simulink model "peacockElettricaSimulink2025b"  (R2025b)
settings: Solver=FixedStepAuto  StopTime=30  FixedStep=0.001  MaxStep=0.001
InitFcn:
  | run('setupParams.m');
StopFcn:
  | plot(out.X, out.Y); axis equal; grid on;
model workspace: external: MATLAB File (data not in the file)
values from neighbouring files (symbols this model uses):
  air_temp = 300    [setupParams.m]    (also in setupParamsSingle.m)
  brake_bias_f = 0.60    (= 0.6)    [setupParams.m]    (also in setupParamsSingle.m)
  brake_bias_r = 1 - brake_bias_f    (= 0.4)    [setupParams.m]    (also in setupParamsSingle.m)
  camber_front = -1.5    [setupParams.m]    (also in setupParamsSingle.m)
  camber_rear = -1    [setupParams.m]    (also in setupParamsSingle.m)
  g = 9.81    [setupParams.m]    (also in setupParamsSingle.m)
  gnd_displ = 0.0    (= 0)    [setupParams.m]    (also in setupParamsSingle.m)
  Kus = 0.00    (= 0)    [setupParams.m]    (also in setupParamsSingle.m)
  l_f = 0.775    [setupParams.m]    (also in setupParamsSingle.m)
  l_r = 0.775    [setupParams.m]    (also in setupParamsSingle.m)
  launch_ramp_rate = 1000.0    (= 1000)    [setupParams.m]    (also in setupParamsSingle.m)
  launch_V_thresh = 5.0    (= 5)    [setupParams.m]    (also in setupParamsSingle.m)
  mass = 300    [setupParams.m]    (also in setupParamsSingle.m)
  mu = 1.5    [setupParams.m]    (also in setupParamsSingle.m)
  nominal_ramp_rate = 1000.0    (= 1000)    [setupParams.m]    (also in setupParamsSingle.m)
  pa_front_wheel = 82700    [setupParams.m]    (also in setupParamsSingle.m)
  pa_rear_wheel = 82700    [setupParams.m]    (also in setupParamsSingle.m)
  pedal_bp = (0:10:100)'    [setupParams.m]    (also in setupParamsSingle.m)
  pedal_map = (pedal_bp / 100) .^ pedal_alpha    [setupParams.m]    (also in setupParamsSingle.m = (pedal_bp / 100) .^ pedal_alpha.Value)
  R_wheel = 0.2032    [setupParams.m]    (also in setupParamsSingle.m)
  regen_I_cont_A = 14.0    (= 14)    [setupParams.m]    (also in setupParamsSingle.m)
  regen_I_peak_A = 21.0    (= 21)    [setupParams.m]    (also in setupParamsSingle.m)
  regen_I_peak_dur_s = 4.0    (= 4)    [setupParams.m]    (also in setupParamsSingle.m)
  regen_P_batt_max_W = 35000    [setupParams.m]    (also in setupParamsSingle.m)
  regen_pedal_thr = 10.0    (= 10)    [setupParams.m]    (also in setupParamsSingle.m)
  regen_speed_crit_rpm = 2000    [setupParams.m]    (also in setupParamsSingle.m = 500)
  regen_speed_min_rpm = 4000    [setupParams.m]    (also in setupParamsSingle.m = 3000)
  regen_T_max = 5    [setupParams.m]    (also in setupParamsSingle.m = Simulink.Parameter(T_rated.Value/2))
  rid_eff = 0.80    (= 0.8)    [setupParams.m]    (also in setupParamsSingle.m)
  rid_ratio = 15    [setupParams.m]    (also in setupParamsSingle.m)
  scale_factor_front = ones(27, 1)    [setupParams.m]    (also in setupParamsSingle.m)
  scale_factor_rear = ones(27, 1)    [setupParams.m]    (also in setupParamsSingle.m)
  slc_Ki = 0    [setupParams.m]    (also in setupParamsSingle.m = Simulink.Parameter(0))
  slc_Kp = 0    [setupParams.m]    (also in setupParamsSingle.m = Simulink.Parameter(0))
  slc_low_sat = -T_peak    (= -21)    [setupParams.m]    (also in setupParamsSingle.m)
  slc_up_sat = T_peak    (= 21)    [setupParams.m]    (also in setupParamsSingle.m)
  slip_bc_coeff = 10    [setupParams.m]    (also in setupParamsSingle.m = Simulink.Parameter(1.5))
  slip_filt_N = 80    [setupParams.m]    (also in setupParamsSingle.m = 15)
  slip_Kd = 0.8    [setupParams.m]    (also in setupParamsSingle.m = Simulink.Parameter(5.0))
  slip_Ki = 13.0    (= 13)    [setupParams.m]    (also in setupParamsSingle.m = Simulink.Parameter(110.0))
  slip_Kp = 50.0    (= 50)    [setupParams.m]    (also in setupParamsSingle.m = Simulink.Parameter(180.0))
  slip_low_sat = 0.0    (= 0)    [setupParams.m]    (also in setupParamsSingle.m)
  slip_ref = 0.15    [setupParams.m]    (also in setupParamsSingle.m = Simulink.Parameter(0.15))
  slip_up_sat = 18    [setupParams.m]    (also in setupParamsSingle.m = 21)
  slip_V_min = 3    [setupParams.m]    (also in setupParamsSingle.m = 1)
  steer_ratio = 4.2    [pure_pursuit.m]    (also in setupParams.m; setupParamsSingle.m)
  T_headroom_max = 3.0    (= 3)    [setupParams.m]    (also in setupParamsSingle.m = Simulink.Parameter(5.0))
  T_peak = 21    [setupParams.m]    (also in setupParamsSingle.m)
  T_rated = 9.8    [setupParams.m]    (also in setupParamsSingle.m = Simulink.Parameter(9.8))
  track_width = (track_width_r + track_width_f)/2    (= 1.2)    [setupParams.m]    (also in setupParamsSingle.m = sqrt(track_width_r^2 + track_width_f^2))
  track_width_f = 1.2    [setupParams.m]    (also in setupParamsSingle.m)
  track_width_r = 1.2    [setupParams.m]    (also in setupParamsSingle.m)
  Ts = 0.01    [setupParams.m]    (also in setupParamsSingle.m)
  tvc_D_thresh = 0.060    (= 0.06)    [setupParams.m]    (also in setupParamsSingle.m)
  tvc_D_thresh_off = 0.03    [setupParams.m]    (also in setupParamsSingle.m)
  tvc_Kd = 8    [setupParams.m]    (also in setupParamsSingle.m = Simulink.Parameter(5))
  tvc_Ki = 250    [setupParams.m]    (also in setupParamsSingle.m = Simulink.Parameter(10))
  tvc_Kp = 650    [setupParams.m]    (also in setupParamsSingle.m = Simulink.Parameter(70))
  tvc_low_sat = Simulink.Parameter(0)    [setupParamsSingle.m]
  tvc_throttle_on = 3.0    (= 3)    [setupParams.m]    (also in setupParamsSingle.m = Simulink.Parameter(3.0))
  tvc_up_sat = Simulink.Parameter(T_peak)    [setupParamsSingle.m]
  tvc_V_off = 2.0    (= 2)    [setupParams.m]    (also in setupParamsSingle.m = Simulink.Parameter(2.0))
  tvc_V_on = 4.0    (= 4)    [setupParams.m]    (also in setupParamsSingle.m = Simulink.Parameter(4.0))
  tvc_yaw_thresh = 0.08    [setupParams.m]    (also in setupParamsSingle.m)
  tvc_yaw_thresh_off = 0.04    [setupParams.m]    (also in setupParamsSingle.m)
  v0_speed = 0.00    (= 0)    [setupParams.m]    (also in setupParamsSingle.m)
  V_dc = 540    [setupParams.m]    (also in setupParamsSingle.m)
  w_engine = 0.005    [setupParams.m]    (also in setupParamsSingle.m)
  wheelbase = l_f + l_r    (= 1.55)    [setupParams.m]    (also in setupParamsSingle.m)
libraries: simulink x12, slpidlib x4, vehdynlibtire x4, vehdynlibsteering x1, sim3dlib x1, sim3dautolib x1, autolibshared x1
(part 2 of 3)

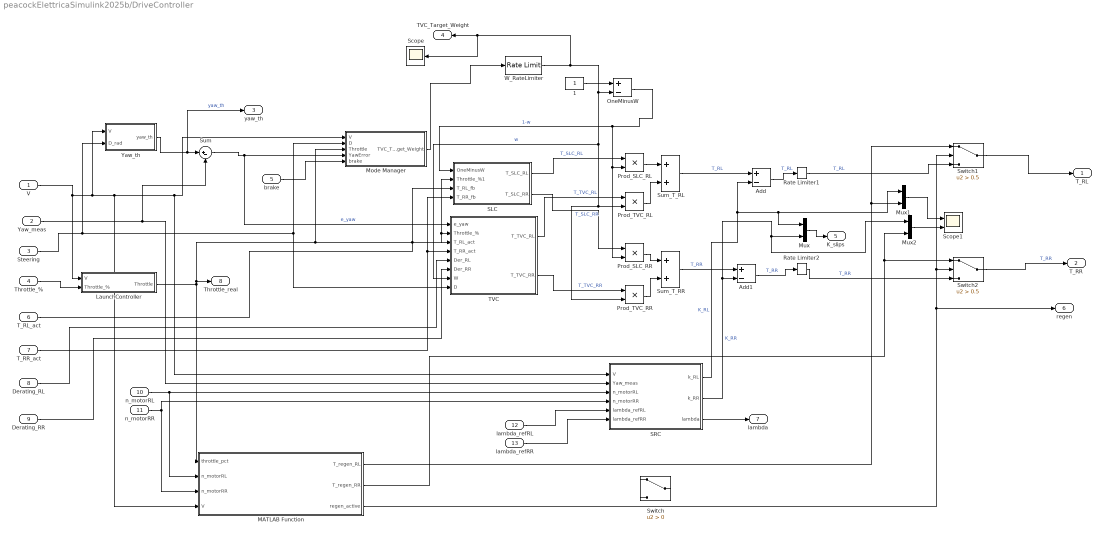
== system peacockElettricaSimulink2025b/DriveController ==
  V : Inport
  Yaw_meas : Inport  Port=2
  Steering : Inport  Port=3
  Throttle_% : Inport  Port=4
  brake : Inport  Port=5
  T_RL_act : Inport  Port=6
  T_RR_act : Inport  Port=7
  Derating_RL : Inport  Port=8
  Derating_RR : Inport  Port=9
  n_motorRL : Inport  Port=10
  n_motorRR : Inport  Port=11
  lambda_refRL : Inport  Port=12
  lambda_refRR : Inport  Port=13
  1 : Constant
  Add : Sum  Inputs=+-
  Add1 : Sum  Inputs=+-
  LaunchController : Subsystem
  MATLAB Function : MATLAB Function  TreatAsAtomicUnit=on
  Mode Manager : Stateflow chart  TreatAsAtomicUnit=on
  Mux : Mux  Inputs=2
  Mux1 : Mux  Inputs=2
  Mux2 : Mux  Inputs=2
  OneMinusW : Sum  Inputs=+-
  Prod_SLC_RL : Product  Inputs=**
  Prod_SLC_RR : Product  Inputs=**
  Prod_TVC_RL : Product  Inputs=**
  Prod_TVC_RR : Product  Inputs=**
  Rate Limiter1 : RateLimiter  RisingSlewLimit=18  FallingSlewLimit=-21  SampleTimeMode=inherited
  Rate Limiter2 : RateLimiter  RisingSlewLimit=18  FallingSlewLimit=-21  SampleTimeMode=inherited
  SLC : Subsystem  TreatAsAtomicUnit=on
  SRC : Subsystem
  Scope : Scope
      settings: ActiveDisplayYMinimum=0.75000000000000011  ActiveDisplayYMaximum=3.25  DataLoggingVariableName=ScopeData5
  Scope1 : Scope  NumInputPorts=2
      settings: ActiveDisplayYMinimum=-0.12499999999999997  ActiveDisplayYMaximum=1.125  DataLoggingVariableName=ScopeData7
  Sum : Sum  Inputs=|+-
  Sum_T_RL : Sum
  Sum_T_RR : Sum
  Switch : Switch  Criteria=u2 > Threshold  SaturateOnIntegerOverflow=off  InputSameDT=off
  Switch1 : Switch  Criteria=u2 > Threshold  Threshold=0.5  SaturateOnIntegerOverflow=off  InputSameDT=off
  Switch2 : Switch  Criteria=u2 > Threshold  Threshold=0.5  SaturateOnIntegerOverflow=off  InputSameDT=off
  TVC : Subsystem
  W_RateLimiter : RateLimiter  RisingSlewLimit=2  FallingSlewLimit=-2  SampleTimeMode=inherited
  Yaw_th : Subsystem
  T_RL : Outport
  T_RR : Outport  Port=2
  yaw_th : Outport  Port=3
  TVC_Target_Weight : Outport  Port=4
  K_slips : Outport  Port=5
  regen : Outport  Port=6
  lambda : Outport  Port=7
  Throttle_real : Outport  Port=8
  wires:
  Steering/1 -> TVC/8(D), Mode Manager/2(D), Yaw_th/2(D_rad)
  Yaw_th/1(yaw_th) -> yaw_th/1, Sum/1  "yaw_th"
  Derating_RL/1 -> TVC/5(Der_RL)
  Yaw_meas/1 -> SRC/2(Yaw_meas), Sum/2
  Derating_RR/1 -> TVC/6(Der_RR)
  LaunchController/1(Throttle) -> Throttle_real/1, Mode Manager/3(Throttle), SLC/2(Throttle_%1), TVC/2(Throttle_%), MATLAB Function/1(throttle_pct)
  TVC/2(T_TVC_RR) -> Prod_TVC_RR/1  "T_TVC_RR"
  V/1 -> LaunchController/1(V), MATLAB Function/4(V), SRC/1(V), Mode Manager/1(V), Yaw_th/1(V)
  T_RL_act/1 -> SLC/3(T_RL_fb), TVC/3(T_RL_act)
  T_RR_act/1 -> SLC/4(T_RR_fb), TVC/4(T_RR_act)
  TVC/1(T_TVC_RL) -> Prod_TVC_RL/1  "T_TVC_RL"
  SLC/1(T_SLC_RL) -> Prod_SLC_RL/1  "T_SLC_RL"
  SLC/2(T_SLC_RR) -> Prod_SLC_RR/1  "T_SLC_RR"
  brake/1 -> Mode Manager/5(brake)
  Sum/1 -> TVC/1(e_yaw), Mode Manager/4(YawError)  "e_yaw"
  W_RateLimiter/1 -> Scope/1, TVC_Target_Weight/1, Prod_TVC_RR/2, Prod_TVC_RL/2, TVC/7(W), OneMinusW/2  "w"
  1/1 -> OneMinusW/1
  OneMinusW/1 -> Prod_SLC_RL/2, Prod_SLC_RR/2, SLC/1(OneMinusW)  "1-w"
  Prod_SLC_RL/1 -> Sum_T_RL/1
  Prod_TVC_RL/1 -> Sum_T_RL/2
  Prod_SLC_RR/1 -> Sum_T_RR/1
  Prod_TVC_RR/1 -> Sum_T_RR/2
  Mode Manager/1(TVC_Target_Weight) -> W_RateLimiter/1
  Add/1 -> Rate Limiter1/1  "T_RL"
  Sum_T_RR/1 -> Add1/1  "T_RR"
  Rate Limiter1/1 -> Switch1/3  "T_RL"
  Add1/1 -> Rate Limiter2/1  "T_RR"
  n_motorRL/1 -> SRC/3(n_motorRL), MATLAB Function/2(n_motorRL)
  n_motorRR/1 -> SRC/4(n_motorRR), MATLAB Function/3(n_motorRR)
  lambda_refRL/1 -> SRC/5(lambda_refRL)
  lambda_refRR/1 -> SRC/6(lambda_refRR)
  SRC/1(k_RL) -> Add/2, Mux/1, Mux1/1  "K_RL"
  SRC/2(k_RR) -> Add1/2, Mux2/1, Mux/2  "K_RR"
  Switch2/1 -> T_RR/1  "T_RR"
  Sum_T_RL/1 -> Add/1  "T_RL"
  Mux/1 -> K_slips/1
  MATLAB Function/2(T_regen_RR) -> Mux2/2, Switch2/1
  MATLAB Function/1(T_regen_RL) -> Switch1/1, Mux1/2
  Mux1/1 -> Scope1/1
  Mux2/1 -> Scope1/2
  MATLAB Function/3(regen_active) -> regen/1, Switch1/2, Switch2/2
  Switch1/1 -> T_RL/1
  Rate Limiter2/1 -> Switch2/3  "T_RR"
  Throttle_%/1 -> LaunchController/2(Throttle_%)
  SRC/3(lambda) -> lambda/1

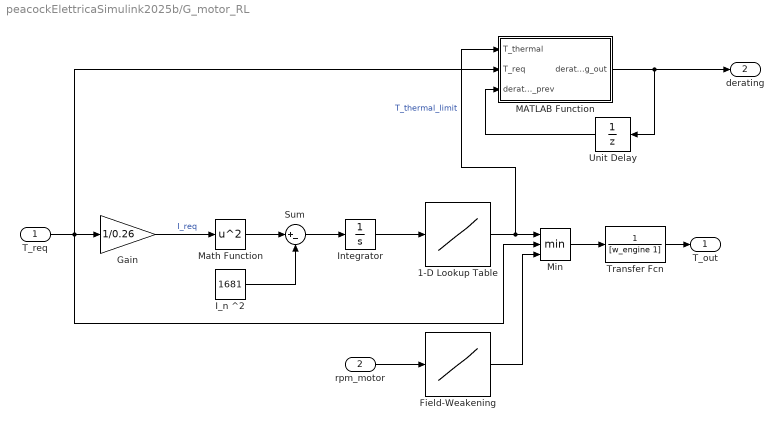
== system peacockElettricaSimulink2025b/G_motor_RL ==
  T_req : Inport
  rpm_motor : Inport  Port=2
  1-D Lookup Table : Lookup_n-D  NumberOfTableDimensions=1  BreakpointsForDimension1=[0, 9268, 11586.6]  Table=[21, 21, 9.8]  InternalRulePriority=Speed  RndMeth=Simplest
  Field-Weakening : Lookup_n-D  NumberOfTableDimensions=1  BreakpointsForDimension1=[0, 12000, 14000, 16000, 18000, 20000]  Table=[21, 21, 20, 16, 9, 0]  InternalRulePriority=Speed  RndMeth=Simplest
  Gain : Gain  Gain=1/0.26
  I_n ^2 : Constant  Value=1681
  Integrator : Integrator  LimitOutput=on  UpperSaturationLimit=11586.6  LowerSaturationLimit=0
  MATLAB Function : MATLAB Function  TreatAsAtomicUnit=on
  Math Function : Math  Operator=square
  Min : MinMax  Inputs=3
  Sum : Sum  Inputs=|+-
  Transfer Fcn : TransferFcn  Denominator=[w_engine 1]
  Unit Delay : UnitDelay  SampleTime=-1
  T_out : Outport
  derating : Outport  Port=2
  wires:
  Sum/1 -> Integrator/1
  I_n ^2/1 -> Sum/2
  Gain/1 -> Math Function/1  "I_req"
  Math Function/1 -> Sum/1
  Integrator/1 -> 1-D Lookup Table/1
  Min/1 -> Transfer Fcn/1
  Transfer Fcn/1 -> T_out/1
  1-D Lookup Table/1 -> MATLAB Function/1(T_thermal), Min/1  "T_thermal_limit"
  T_req/1 -> MATLAB Function/2(T_req), Min/2, Gain/1
  MATLAB Function/1(derating_out) -> Unit Delay/1, derating/1
  Unit Delay/1 -> MATLAB Function/3(derating_prev)
  rpm_motor/1 -> Field-Weakening/1
  Field-Weakening/1 -> Min/3

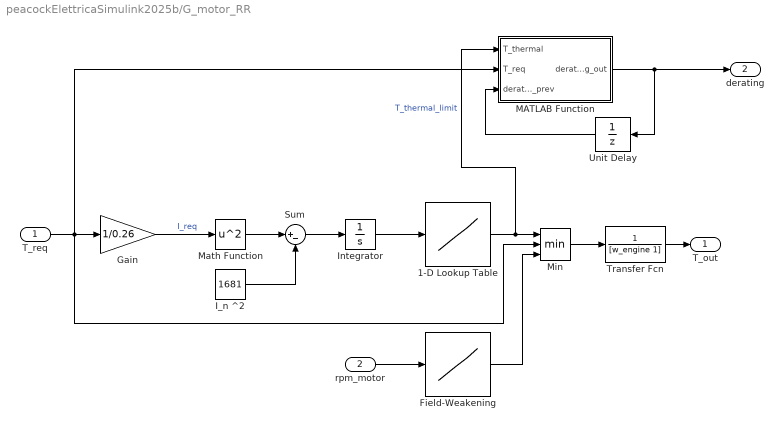
== system peacockElettricaSimulink2025b/G_motor_RR ==
  T_req : Inport
  rpm_motor : Inport  Port=2
  1-D Lookup Table : Lookup_n-D  NumberOfTableDimensions=1  BreakpointsForDimension1=[0, 9268, 11586.6]  Table=[21, 21, 9.8]  InternalRulePriority=Speed  RndMeth=Simplest
  Field-Weakening : Lookup_n-D  NumberOfTableDimensions=1  BreakpointsForDimension1=[0, 12000, 14000, 16000, 18000, 20000]  Table=[21, 21, 20, 16, 9, 0]  InternalRulePriority=Speed  RndMeth=Simplest
  Gain : Gain  Gain=1/0.26
  I_n ^2 : Constant  Value=1681
  Integrator : Integrator  LimitOutput=on  UpperSaturationLimit=11586.6  LowerSaturationLimit=0
  MATLAB Function : MATLAB Function  TreatAsAtomicUnit=on
  Math Function : Math  Operator=square
  Min : MinMax  Inputs=3
  Sum : Sum  Inputs=|+-
  Transfer Fcn : TransferFcn  Denominator=[w_engine 1]
  Unit Delay : UnitDelay  SampleTime=-1
  T_out : Outport
  derating : Outport  Port=2
  wires:
  Sum/1 -> Integrator/1
  I_n ^2/1 -> Sum/2
  Gain/1 -> Math Function/1  "I_req"
  Math Function/1 -> Sum/1
  Integrator/1 -> 1-D Lookup Table/1
  Min/1 -> Transfer Fcn/1
  Transfer Fcn/1 -> T_out/1
  1-D Lookup Table/1 -> MATLAB Function/1(T_thermal), Min/1  "T_thermal_limit"
  T_req/1 -> MATLAB Function/2(T_req), Min/2, Gain/1
  MATLAB Function/1(derating_out) -> Unit Delay/1, derating/1
  Unit Delay/1 -> MATLAB Function/3(derating_prev)
  rpm_motor/1 -> Field-Weakening/1
  Field-Weakening/1 -> Min/3

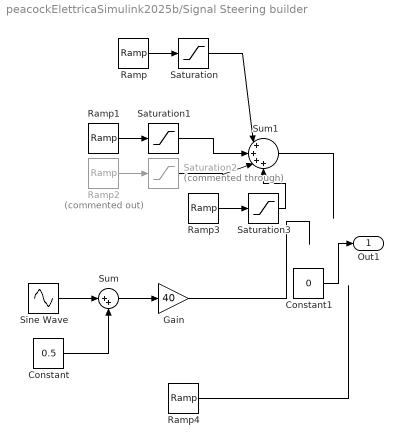
== system peacockElettricaSimulink2025b/Signal Steering builder ==
  Constant : Constant  Value=0.5
  Constant1 : Constant  Value=0
  Gain : Gain  Gain=40
  Ramp : simulink/Sources/Ramp  slope=20  start=0  InitialOutput=0
  Ramp1 : simulink/Sources/Ramp  slope=-20  start=30  InitialOutput=0
  Ramp2 : simulink/Sources/Ramp  Commented=on  slope=-20  start=14  InitialOutput=0
  Ramp3 : simulink/Sources/Ramp  slope=20  start=22  InitialOutput=0
  Ramp4 : simulink/Sources/Ramp  slope=30  start=4  InitialOutput=0
  Saturation : Saturate  UpperLimit=40  LowerLimit=-40
  Saturation1 : Saturate  UpperLimit=40  LowerLimit=-40
  Saturation2 : Saturate  Commented=through  UpperLimit=40  LowerLimit=-40
  Saturation3 : Saturate  UpperLimit=40  LowerLimit=-40
  Sine Wave : Sin  Amplitude=0.5  Frequency=0.3  SampleTime=0.2
  Sum : Sum  Inputs=|++
  Sum1 : Sum  Inputs=|++++
  Out1 : Outport
  wires:
  Ramp/1 -> Saturation/1
  Ramp1/1 -> Saturation1/1
  Ramp2/1 -> Saturation2/1
  Ramp3/1 -> Saturation3/1
  Saturation3/1 -> Sum1/4
  Saturation/1 -> Sum1/1
  Saturation1/1 -> Sum1/2
  Saturation2/1 -> Sum1/3
  Sum1/1 -> ?
  Constant/1 -> Sum/2
  Sine Wave/1 -> Sum/1
  Sum/1 -> Gain/1
  Gain/1 -> ?
  Ramp4/1 -> ?
  Constant1/1 -> Out1/1

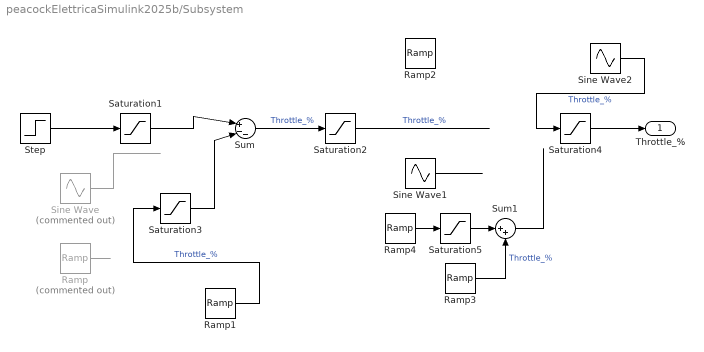
== system peacockElettricaSimulink2025b/Subsystem ==
  Ramp : simulink/Sources/Ramp  Commented=on  slope=1  start=0  InitialOutput=0
  Ramp1 : simulink/Sources/Ramp  slope=40  start=10  InitialOutput=0
  Ramp2 : simulink/Sources/Ramp  slope=100  start=2  InitialOutput=0
  Ramp3 : simulink/Sources/Ramp  slope=50  start=2  InitialOutput=0
  Ramp4 : simulink/Sources/Ramp  slope=50  start=0  InitialOutput=0
  Saturation1 : Saturate  UpperLimit=100  LowerLimit=0
  Saturation2 : Saturate  UpperLimit=100  LowerLimit=0
  Saturation3 : Saturate  UpperLimit=40  LowerLimit=0
  Saturation4 : Saturate  UpperLimit=100  LowerLimit=0
  Saturation5 : Saturate  UpperLimit=60  LowerLimit=0
  Sine Wave : Sin  Commented=on  Amplitude=150  Frequency=0.5  SampleTime=0.2
  Sine Wave1 : Sin  Amplitude=30  Frequency=4  SampleTime=0.01
  Sine Wave2 : Sin  Amplitude=800  Frequency=0.3  SampleTime=Ts
  Step : Step  After=100  SampleTime=0
  Sum : Sum  Inputs=|+--
  Sum1 : Sum  Inputs=|++
  Throttle_% : Outport
  wires:
  Step/1 -> Saturation1/1
  Sine Wave/1 -> ?
  Ramp1/1 -> Saturation3/1  "Throttle_%"
  Ramp/1 -> ?
  Saturation1/1 -> Sum/1
  Saturation3/1 -> Sum/2
  Sum/1 -> Saturation2/1  "Throttle_%"
  Sine Wave2/1 -> Saturation4/1  "Throttle_%"
  Saturation2/1 -> ?  "Throttle_%"
  Ramp3/1 -> Sum1/2  "Throttle_%"
  Sine Wave1/1 -> ?
  Sum1/1 -> ?
  Ramp4/1 -> Saturation5/1
  Saturation4/1 -> Throttle_%/1
  Saturation5/1 -> Sum1/1

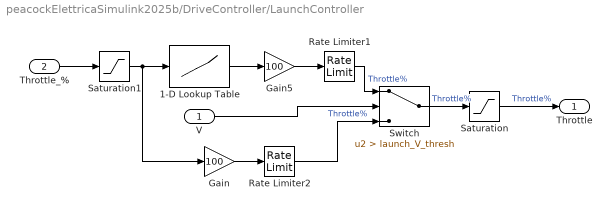
== system peacockElettricaSimulink2025b/DriveController/LaunchController ==
  V : Inport
  Throttle_% : Inport  Port=2
  1-D Lookup Table : Lookup_n-D  NumberOfTableDimensions=1  BreakpointsForDimension1=pedal_bp  Table=pedal_map  ExtrapMethod=Clip  UseLastTableValue=on  InternalRulePriority=Speed  RndMeth=Simplest
  Gain : Gain  Gain=100
  Gain5 : Gain  Gain=100
  Rate Limiter1 : RateLimiter  RisingSlewLimit=launch_ramp_rate  FallingSlewLimit=-100  SampleTimeMode=inherited
  Rate Limiter2 : RateLimiter  RisingSlewLimit=nominal_ramp_rate  FallingSlewLimit=-100  SampleTimeMode=inherited
  Saturation : Saturate  UpperLimit=100  LowerLimit=0
  Saturation1 : Saturate  UpperLimit=100  LowerLimit=0
  Switch : Switch  Criteria=u2 > Threshold  Threshold=launch_V_thresh  SaturateOnIntegerOverflow=off  InputSameDT=off
  Throttle : Outport
  wires:
  Throttle_%/1 -> Saturation1/1
  Saturation1/1 -> Gain/1, 1-D Lookup Table/1
  1-D Lookup Table/1 -> Gain5/1
  Gain5/1 -> Rate Limiter1/1
  Saturation/1 -> Throttle/1  "Throttle%"
  Gain/1 -> Rate Limiter2/1
  Rate Limiter2/1 -> Switch/3  "Throttle%"
  Rate Limiter1/1 -> Switch/1  "Throttle%"
  V/1 -> Switch/2
  Switch/1 -> Saturation/1  "Throttle%"

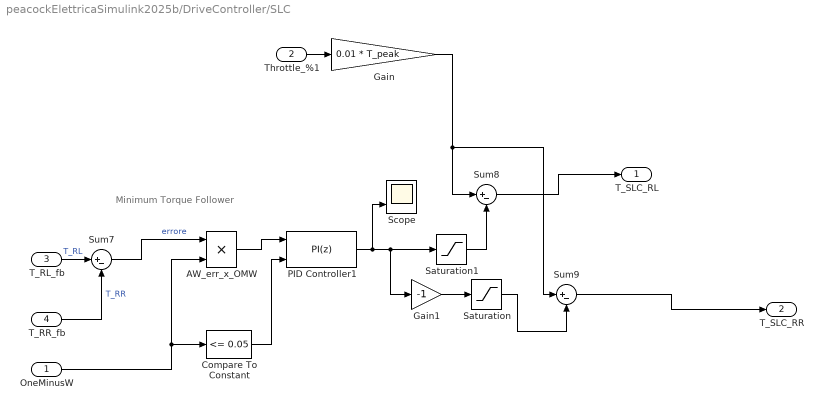
== system peacockElettricaSimulink2025b/DriveController/SLC ==
  note: Minimum Torque Follower
  OneMinusW : Inport
  Throttle_%1 : Inport  Port=2
  T_RL_fb : Inport  Port=3
  T_RR_fb : Inport  Port=4
  AW_err_x_OMW : Product  Inputs=**
  Compare To Constant : simulink/Logic and Bit Operations/Compare To Constant  relop=<=  const=0.05  OutDataTypeStr=boolean
  Gain : Gain  Gain=0.01 * T_peak
  Gain1 : Gain  Gain=-1
  PID Controller1 : slpidlib/PID Controller  Controller=PI  Form=Parallel  TimeDomain=Discrete-time  UseExternalTs=off  SampleTime=Ts  IntegratorMethod=Forward Euler  FilterMethod=Forward Euler  ControllerParametersSource=internal  P=slc_Kp  I=slc_Ki  UseKiTs=off  D=0  UseExternalDerivativeSource=off  N=100  UseFilter=off  TunerSelectOption=Transfer Function Based (PID Tuner App)  InitialConditionSource=internal  InitialConditionForIntegrator=0  InitialConditionForFilter=0  DifferentiatorICPrevScaledInput=0  ExternalReset=level  TrackingMode=off  Kt=1  LimitOutput=on  SatLimitsSource=internal  UpperSaturationLimit=slc_up_sat  LowerSaturationLimit=slc_low_sat  LinearizeAsGain=on  AntiWindupMode=back-calculation  Kb=1  LimitIntegrator=off  UpperIntegratorSaturationLimit=inf  LowerIntegratorSaturationLimit=-inf  POutMin=[]  POutMax=[]  IOutMin=[]  IOutMax=[]  DOutMin=[]  DOutMax=[]  NOutMin=[]  NOutMax=[]  SumOutMin=[]  SumOutMax=[]  SaturationOutMin=[]  SaturationOutMax=[]  PParamMin=[]  PParamMax=[]  IParamMin=[]  IParamMax=[]  DParamMin=[]  DParamMax=[]  NParamMin=[]  NParamMax=[]  KbParamMin=[]  KbParamMax=[]  KtParamMin=[]  KtParamMax=[]  KbOutMin=[]  KbOutMax=[]  KtOutMin=[]  KtOutMax=[]  IntegratorOutMin=[]  IntegratorOutMax=[]  FilterOutMin=[]  FilterOutMax=[]  SumI1OutMin=[]  SumI1OutMax=[]  SumI2OutMin=[]  SumI2OutMax=[]  SumI3OutMin=[]  SumI3OutMax=[]  SumI4OutMin=[]  SumI4OutMax=[]  SumDOutMin=[]  SumDOutMax=[]  DifferentiatorOutMin=[]  DifferentiatorOutMax=[]  FilterDiffOutCoefMin=[]  FilterDiffOutCoefMax=[]  ReciprocalOutMin=[]  ReciprocalOutMax=[]  SumDenOutMin=[]  SumDenOutMax=[]  SumNumOutMin=[]  SumNumOutMax=[]  DivideOutMin=[]  DivideOutMax=[]  UdiffTsProdOutMin=[]  UdiffTsProdOutMax=[]  NTsProdOutMin=[]  NTsProdOutMax=[]  UintegralTsProdOutMin=[]  UintegralTsProdOutMax=[]  UngainTsProdOutMin=[]  UngainTsProdOutMax=[]  ClampingZeroOutDataTypeStr=Inherit: Inherit via back propagation  ClampingZeroOutMin=[]  ClampingZeroOutMax=[]  FilterDenConstantOutDataTypeStr=Inherit: Inherit via back propagation  FilterDenConstantOutMin=[]  FilterDenConstantOutMax=[]  PCopyOutDataTypeStr=Inherit: Inherit via back propagation  PCopyOutMin=[]  PCopyOutMax=[]  NCopyOutDataTypeStr=Inherit: Inherit via back propagation  NCopyOutMin=[]  NCopyOutMax=[]  IntegratorContinuousStateAttributes=''  IntegratorStateMustResolveToSignalObject=off  IntegratorRTWStateStorageClass=Auto  FilterContinuousStateAttributes=''  FilterStateMustResolveToSignalObject=off  FilterRTWStateStorageClass=Auto  ParallelPVariant=InternalParameters  IdealPVariant=Disabled  IVariant=InternalParameters  DVariant=Disabled  IntegratorVariant=Discrete  SatVariant=Enabled  AWVariant=BackCalculation  PCopyVariant=Disabled  TRVariant=Disabled  FdbkBlocksVariant=Forward  IdealPFdbkVariant=Disabled  SatFdbkVariant=Disabled  DerivativeFilterVariant=Disabled  NVariant=Disabled  NCopyVariant=Disabled_SignalSpec  FilterICVariant=Disabled  IntegratorICVariant=InternalICs  ExternalResetVariant=ExternalReset  TRSumVariant=Passthrough  SumFdbkVariant=Disabled  SumVariant=Sum_PI  TsampFilterVariant=InternalTs  TsampNgainVariant=Passthrough  TsampIntegralVariant=Disabled_SignalSpec  ExternalSaturationOutDataTypeStr=Inherit: Same as second input  DerivativeSourceVariant=Disabled  PreIntVariant=InternalPreInt
  Saturation : Saturate  UpperLimit=inf  LowerLimit=0
  Saturation1 : Saturate  UpperLimit=inf  LowerLimit=0
  Scope : Scope  NumInputPorts=2
      settings: ActiveDisplayYMinimum=-14.980593372573752  ActiveDisplayYMaximum=14.997843708063737
  Sum7 : Sum  Inputs=|+-
  Sum8 : Sum  Inputs=|+-
  Sum9 : Sum  Inputs=|+-
  T_SLC_RL : Outport
  T_SLC_RR : Outport  Port=2
  wires:
  T_RL_fb/1 -> Sum7/1  "T_RL"
  T_RR_fb/1 -> Sum7/2  "T_RR"
  Gain/1 -> Sum8/1, Sum9/1
  PID Controller1/1 -> Saturation1/1, Gain1/1, Scope/2
  Sum8/1 -> T_SLC_RL/1
  Gain1/1 -> Saturation/1
  Saturation/1 -> Sum9/2
  Sum9/1 -> T_SLC_RR/1
  Saturation1/1 -> Sum8/2
  Throttle_%1/1 -> Gain/1
  Sum7/1 -> AW_err_x_OMW/1  "errore"
  OneMinusW/1 -> Compare To Constant/1, AW_err_x_OMW/2
  AW_err_x_OMW/1 -> PID Controller1/1
  Compare To Constant/1 -> PID Controller1/2

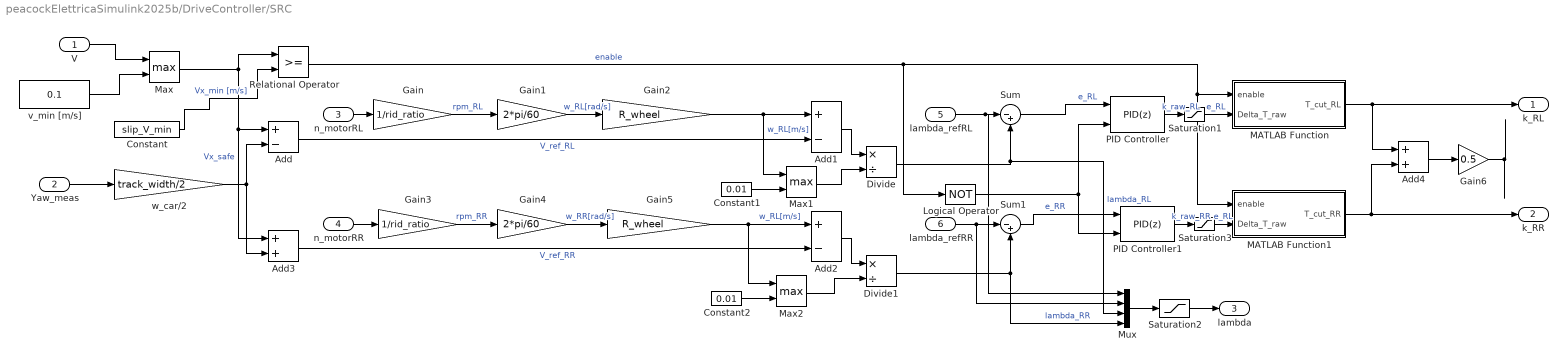
== system peacockElettricaSimulink2025b/DriveController/SRC ==
  V : Inport
  Yaw_meas : Inport  Port=2
  n_motorRL : Inport  Port=3
  n_motorRR : Inport  Port=4
  lambda_refRL : Inport  Port=5
  lambda_refRR : Inport  Port=6
  Add : Sum  Inputs=+-
  Add1 : Sum  Inputs=+-
  Add2 : Sum  Inputs=+-
  Add3 : Sum
  Add4 : Sum
  Constant : Constant  Value=slip_V_min
  Constant1 : Constant  Value=0.01
  Constant2 : Constant  Value=0.01
  Divide : Product  Inputs=*/
  Divide1 : Product  Inputs=*/
  Gain : Gain  Gain=1/rid_ratio
  Gain1 : Gain  Gain=2*pi/60
  Gain2 : Gain  Gain=R_wheel
  Gain3 : Gain  Gain=1/rid_ratio
  Gain4 : Gain  Gain=2*pi/60
  Gain5 : Gain  Gain=R_wheel
  Gain6 : Gain  Gain=0.5
  Logical Operator : Logic  Operator=NOT  AllPortsSameDT=off  OutDataTypeStr=boolean
  MATLAB Function : MATLAB Function  TreatAsAtomicUnit=on
  MATLAB Function1 : MATLAB Function  TreatAsAtomicUnit=on
  Max : MinMax  Function=max  Inputs=2
  Max1 : MinMax  Function=max  Inputs=2
  Max2 : MinMax  Function=max  Inputs=2
  Mux : Mux
  PID Controller : slpidlib/PID Controller  Controller=PID  Form=Parallel  TimeDomain=Discrete-time  UseExternalTs=off  SampleTime=Ts  IntegratorMethod=Forward Euler  FilterMethod=Forward Euler  ControllerParametersSource=internal  P=slip_Kp  I=slip_Ki  UseKiTs=off  D=slip_Kd  UseExternalDerivativeSource=off  N=slip_filt_N  UseFilter=on  TunerSelectOption=Transfer Function Based (PID Tuner App)  InitialConditionSource=internal  InitialConditionForIntegrator=0  InitialConditionForFilter=0  DifferentiatorICPrevScaledInput=0  ExternalReset=level  TrackingMode=off  Kt=1  LimitOutput=on  SatLimitsSource=internal  UpperSaturationLimit=slip_up_sat  LowerSaturationLimit=slip_low_sat  LinearizeAsGain=on  AntiWindupMode=back-calculation  Kb=slip_bc_coeff  LimitIntegrator=off  UpperIntegratorSaturationLimit=inf  LowerIntegratorSaturationLimit=-inf  POutMin=[]  POutMax=[]  IOutMin=[]  IOutMax=[]  DOutMin=[]  DOutMax=[]  NOutMin=[]  NOutMax=[]  SumOutMin=[]  SumOutMax=[]  SaturationOutMin=[]  SaturationOutMax=[]  PParamMin=[]  PParamMax=[]  IParamMin=[]  IParamMax=[]  DParamMin=[]  DParamMax=[]  NParamMin=[]  NParamMax=[]  KbParamMin=[]  KbParamMax=[]  KtParamMin=[]  KtParamMax=[]  KbOutMin=[]  KbOutMax=[]  KtOutMin=[]  KtOutMax=[]  IntegratorOutMin=[]  IntegratorOutMax=[]  FilterOutMin=[]  FilterOutMax=[]  SumI1OutMin=[]  SumI1OutMax=[]  SumI2OutMin=[]  SumI2OutMax=[]  SumI3OutMin=[]  SumI3OutMax=[]  SumI4OutMin=[]  SumI4OutMax=[]  SumDOutMin=[]  SumDOutMax=[]  DifferentiatorOutMin=[]  DifferentiatorOutMax=[]  FilterDiffOutCoefMin=[]  FilterDiffOutCoefMax=[]  ReciprocalOutMin=[]  ReciprocalOutMax=[]  SumDenOutMin=[]  SumDenOutMax=[]  SumNumOutMin=[]  SumNumOutMax=[]  DivideOutMin=[]  DivideOutMax=[]  UdiffTsProdOutMin=[]  UdiffTsProdOutMax=[]  NTsProdOutMin=[]  NTsProdOutMax=[]  UintegralTsProdOutMin=[]  UintegralTsProdOutMax=[]  UngainTsProdOutMin=[]  UngainTsProdOutMax=[]  ClampingZeroOutDataTypeStr=Inherit: Inherit via back propagation  ClampingZeroOutMin=[]  ClampingZeroOutMax=[]  FilterDenConstantOutDataTypeStr=Inherit: Inherit via back propagation  FilterDenConstantOutMin=[]  FilterDenConstantOutMax=[]  PCopyOutDataTypeStr=Inherit: Inherit via back propagation  PCopyOutMin=[]  PCopyOutMax=[]  NCopyOutDataTypeStr=Inherit: Inherit via back propagation  NCopyOutMin=[]  NCopyOutMax=[]  IntegratorContinuousStateAttributes=''  IntegratorStateMustResolveToSignalObject=off  IntegratorRTWStateStorageClass=Auto  FilterContinuousStateAttributes=''  FilterStateMustResolveToSignalObject=off  FilterRTWStateStorageClass=Auto  ParallelPVariant=InternalParameters  IdealPVariant=Disabled  IVariant=InternalParameters  DVariant=InternalParameters  IntegratorVariant=Discrete  SatVariant=Enabled  AWVariant=BackCalculation  PCopyVariant=Disabled  TRVariant=Disabled  FdbkBlocksVariant=Forward  IdealPFdbkVariant=Disabled  SatFdbkVariant=Disabled  DerivativeFilterVariant=ForwardEulerFilter  NVariant=InternalParameters  NCopyVariant=Disabled  FilterICVariant=InternalICsFilter  IntegratorICVariant=InternalICs  ExternalResetVariant=ExternalReset  TRSumVariant=Passthrough  SumFdbkVariant=Disabled  SumVariant=Sum_PID  TsampFilterVariant=InternalTs  TsampNgainVariant=Passthrough  TsampIntegralVariant=Disabled_SignalSpec  ExternalSaturationOutDataTypeStr=Inherit: Same as second input  DerivativeSourceVariant=ErrorSignal  PreIntVariant=InternalPreInt
  PID Controller1 : slpidlib/PID Controller  Controller=PID  Form=Parallel  TimeDomain=Discrete-time  UseExternalTs=off  SampleTime=Ts  IntegratorMethod=Forward Euler  FilterMethod=Forward Euler  ControllerParametersSource=internal  P=slip_Kp  I=slip_Ki  UseKiTs=off  D=slip_Kd  UseExternalDerivativeSource=off  N=slip_filt_N  UseFilter=on  TunerSelectOption=Transfer Function Based (PID Tuner App)  InitialConditionSource=internal  InitialConditionForIntegrator=0  InitialConditionForFilter=0  DifferentiatorICPrevScaledInput=0  ExternalReset=level  TrackingMode=off  Kt=1  LimitOutput=on  SatLimitsSource=internal  UpperSaturationLimit=slip_up_sat  LowerSaturationLimit=slip_low_sat  LinearizeAsGain=on  AntiWindupMode=back-calculation  Kb=slip_bc_coeff  LimitIntegrator=off  UpperIntegratorSaturationLimit=inf  LowerIntegratorSaturationLimit=-inf  POutMin=[]  POutMax=[]  IOutMin=[]  IOutMax=[]  DOutMin=[]  DOutMax=[]  NOutMin=[]  NOutMax=[]  SumOutMin=[]  SumOutMax=[]  SaturationOutMin=[]  SaturationOutMax=[]  PParamMin=[]  PParamMax=[]  IParamMin=[]  IParamMax=[]  DParamMin=[]  DParamMax=[]  NParamMin=[]  NParamMax=[]  KbParamMin=[]  KbParamMax=[]  KtParamMin=[]  KtParamMax=[]  KbOutMin=[]  KbOutMax=[]  KtOutMin=[]  KtOutMax=[]  IntegratorOutMin=[]  IntegratorOutMax=[]  FilterOutMin=[]  FilterOutMax=[]  SumI1OutMin=[]  SumI1OutMax=[]  SumI2OutMin=[]  SumI2OutMax=[]  SumI3OutMin=[]  SumI3OutMax=[]  SumI4OutMin=[]  SumI4OutMax=[]  SumDOutMin=[]  SumDOutMax=[]  DifferentiatorOutMin=[]  DifferentiatorOutMax=[]  FilterDiffOutCoefMin=[]  FilterDiffOutCoefMax=[]  ReciprocalOutMin=[]  ReciprocalOutMax=[]  SumDenOutMin=[]  SumDenOutMax=[]  SumNumOutMin=[]  SumNumOutMax=[]  DivideOutMin=[]  DivideOutMax=[]  UdiffTsProdOutMin=[]  UdiffTsProdOutMax=[]  NTsProdOutMin=[]  NTsProdOutMax=[]  UintegralTsProdOutMin=[]  UintegralTsProdOutMax=[]  UngainTsProdOutMin=[]  UngainTsProdOutMax=[]  ClampingZeroOutDataTypeStr=Inherit: Inherit via back propagation  ClampingZeroOutMin=[]  ClampingZeroOutMax=[]  FilterDenConstantOutDataTypeStr=Inherit: Inherit via back propagation  FilterDenConstantOutMin=[]  FilterDenConstantOutMax=[]  PCopyOutDataTypeStr=Inherit: Inherit via back propagation  PCopyOutMin=[]  PCopyOutMax=[]  NCopyOutDataTypeStr=Inherit: Inherit via back propagation  NCopyOutMin=[]  NCopyOutMax=[]  IntegratorContinuousStateAttributes=''  IntegratorStateMustResolveToSignalObject=off  IntegratorRTWStateStorageClass=Auto  FilterContinuousStateAttributes=''  FilterStateMustResolveToSignalObject=off  FilterRTWStateStorageClass=Auto  ParallelPVariant=InternalParameters  IdealPVariant=Disabled  IVariant=InternalParameters  DVariant=InternalParameters  IntegratorVariant=Discrete  SatVariant=Enabled  AWVariant=BackCalculation  PCopyVariant=Disabled  TRVariant=Disabled  FdbkBlocksVariant=Forward  IdealPFdbkVariant=Disabled  SatFdbkVariant=Disabled  DerivativeFilterVariant=ForwardEulerFilter  NVariant=InternalParameters  NCopyVariant=Disabled  FilterICVariant=InternalICsFilter  IntegratorICVariant=InternalICs  ExternalResetVariant=ExternalReset  TRSumVariant=Passthrough  SumFdbkVariant=Disabled  SumVariant=Sum_PID  TsampFilterVariant=InternalTs  TsampNgainVariant=Passthrough  TsampIntegralVariant=Disabled_SignalSpec  ExternalSaturationOutDataTypeStr=Inherit: Same as second input  DerivativeSourceVariant=ErrorSignal  PreIntVariant=InternalPreInt
  Relational Operator : RelationalOperator  OutDataTypeStr=boolean  RndMeth=Simplest  InputSameDT=off
  Saturation1 : Saturate  UpperLimit=inf  LowerLimit=0
  Saturation2 : Saturate  UpperLimit=1  LowerLimit=0
  Saturation3 : Saturate  UpperLimit=inf  LowerLimit=0
  Sum : Sum  Inputs=|-+
  Sum1 : Sum  Inputs=|-+
  v_min [m/s] : Constant  Value=0.1
  w_car/2 : Gain  Gain=track_width/2
  k_RL : Outport
  k_RR : Outport  Port=2
  lambda : Outport  Port=3
  wires:
  V/1 -> Max/1
  v_min [m/s]/1 -> Max/2
  Max/1 -> Relational Operator/1, Add3/1, Add/1  "Vx_safe"
  Constant/1 -> Relational Operator/2  "Vx_min [m/s]"
  Yaw_meas/1 -> w_car/2/1
  Add/1 -> Add1/2  "V_ref_RL"
  n_motorRL/1 -> Gain/1
  Gain/1 -> Gain1/1  "rpm_RL"
  Add1/1 -> Divide/1
  Divide/1 -> Mux/3, Sum/2  "lambda_RL"
  w_car/2/1 -> Add3/2, Add/2
  Gain1/1 -> Gain2/1  "w_RL[rad/s]"
  Gain2/1 -> Max1/1, Add1/1  "w_RL[m/s]"
  Gain4/1 -> Gain5/1  "w_RR[rad/s]"
  Gain3/1 -> Gain4/1  "rpm_RR"
  Divide1/1 -> Sum1/2, Mux/4  "lambda_RR"
  n_motorRR/1 -> Gain3/1
  Add3/1 -> Add2/2  "V_ref_RR"
  Add2/1 -> Divide1/1
  lambda_refRL/1 -> Mux/1, Sum/1
  Relational Operator/1 -> Logical Operator/1, MATLAB Function1/1(enable), MATLAB Function/1(enable)  "enable"
  PID Controller/1 -> Saturation1/1  "k_raw_RL"
  MATLAB Function/1(T_cut_RL) -> k_RL/1, Add4/1
  PID Controller1/1 -> Saturation3/1  "k_raw_RR"
  lambda_refRR/1 -> Mux/2, Sum1/1
  MATLAB Function1/1(T_cut_RR) -> k_RR/1, Add4/2
  Logical Operator/1 -> PID Controller1/2, PID Controller/2
  Sum1/1 -> PID Controller1/1  "e_RR"
  Sum/1 -> PID Controller/1  "e_RL"
  Max1/1 -> Divide/2
  Constant1/1 -> Max1/2
  Max2/1 -> Divide1/2
  Constant2/1 -> Max2/2
  Gain5/1 -> Max2/1, Add2/1  "w_RL[m/s]"
  Mux/1 -> Saturation2/1
  Saturation2/1 -> lambda/1
  Add4/1 -> Gain6/1
  Gain6/1 -> ?
  Saturation1/1 -> MATLAB Function/2(Delta_T_raw)  "e_RL"
  Saturation3/1 -> MATLAB Function1/2(Delta_T_raw)  "e_RL"

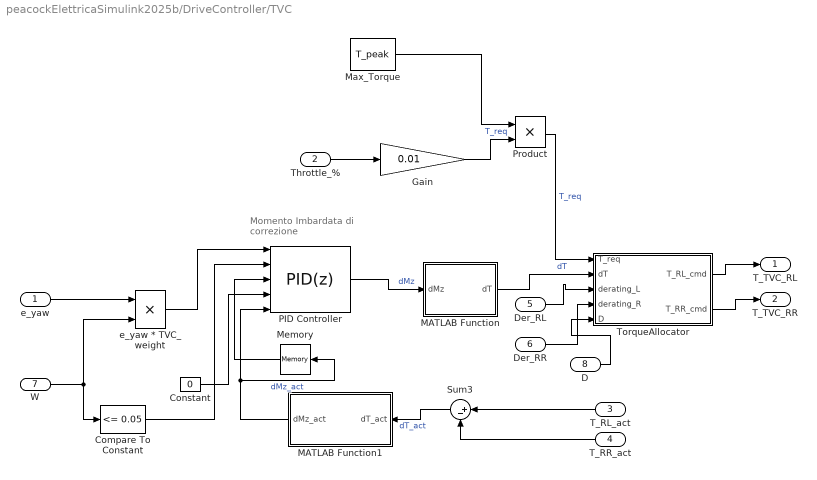
== system peacockElettricaSimulink2025b/DriveController/TVC ==
  note: Momento Imbardata di correzione
  e_yaw : Inport
  Throttle_% : Inport  Port=2
  T_RL_act : Inport  Port=3
  T_RR_act : Inport  Port=4
  Der_RL : Inport  Port=5
  Der_RR : Inport  Port=6
  W : Inport  Port=7
  D : Inport  Port=8
  Compare To Constant : simulink/Logic and Bit Operations/Compare To Constant  relop=<=  const=0.05  OutDataTypeStr=boolean
  Constant : Constant  Value=0
  Gain : Gain  Gain=0.01
  MATLAB Function : MATLAB Function  TreatAsAtomicUnit=on
  MATLAB Function1 : MATLAB Function  TreatAsAtomicUnit=on
  Max_Torque : Constant  Value=T_peak
  Memory : Memory
  PID Controller : slpidlib/PID Controller  Controller=PID  Form=Parallel  TimeDomain=Discrete-time  UseExternalTs=off  SampleTime=0.05  IntegratorMethod=Forward Euler  FilterMethod=Forward Euler  ControllerParametersSource=internal  P=tvc_Kp  I=tvc_Ki  UseKiTs=off  D=tvc_Kd  UseExternalDerivativeSource=off  N=10  UseFilter=on  TunerSelectOption=Transfer Function Based (PID Tuner App)  InitialConditionSource=external  InitialConditionForIntegrator=0  InitialConditionForFilter=0  DifferentiatorICPrevScaledInput=0  ExternalReset=level  TrackingMode=on  Kt=1.6  LimitOutput=on  SatLimitsSource=internal  UpperSaturationLimit=tvc_up_sat  LowerSaturationLimit=tvc_low_sat  LinearizeAsGain=on  AntiWindupMode=back-calculation  Kb=1  LimitIntegrator=off  UpperIntegratorSaturationLimit=inf  LowerIntegratorSaturationLimit=-inf  POutMin=[]  POutMax=[]  IOutMin=[]  IOutMax=[]  DOutMin=[]  DOutMax=[]  NOutMin=[]  NOutMax=[]  SumOutMin=[]  SumOutMax=[]  SaturationOutMin=[]  SaturationOutMax=[]  PParamMin=[]  PParamMax=[]  IParamMin=[]  IParamMax=[]  DParamMin=[]  DParamMax=[]  NParamMin=[]  NParamMax=[]  KbParamMin=[]  KbParamMax=[]  KtParamMin=[]  KtParamMax=[]  KbOutMin=[]  KbOutMax=[]  KtOutMin=[]  KtOutMax=[]  IntegratorOutMin=[]  IntegratorOutMax=[]  FilterOutMin=[]  FilterOutMax=[]  SumI1OutMin=[]  SumI1OutMax=[]  SumI2OutMin=[]  SumI2OutMax=[]  SumI3OutMin=[]  SumI3OutMax=[]  SumI4OutMin=[]  SumI4OutMax=[]  SumDOutMin=[]  SumDOutMax=[]  DifferentiatorOutMin=[]  DifferentiatorOutMax=[]  FilterDiffOutCoefMin=[]  FilterDiffOutCoefMax=[]  ReciprocalOutMin=[]  ReciprocalOutMax=[]  SumDenOutMin=[]  SumDenOutMax=[]  SumNumOutMin=[]  SumNumOutMax=[]  DivideOutMin=[]  DivideOutMax=[]  UdiffTsProdOutMin=[]  UdiffTsProdOutMax=[]  NTsProdOutMin=[]  NTsProdOutMax=[]  UintegralTsProdOutMin=[]  UintegralTsProdOutMax=[]  UngainTsProdOutMin=[]  UngainTsProdOutMax=[]  ClampingZeroOutDataTypeStr=Inherit: Inherit via back propagation  ClampingZeroOutMin=[]  ClampingZeroOutMax=[]  FilterDenConstantOutDataTypeStr=Inherit: Inherit via back propagation  FilterDenConstantOutMin=[]  FilterDenConstantOutMax=[]  PCopyOutDataTypeStr=Inherit: Inherit via back propagation  PCopyOutMin=[]  PCopyOutMax=[]  NCopyOutDataTypeStr=Inherit: Inherit via back propagation  NCopyOutMin=[]  NCopyOutMax=[]  IntegratorContinuousStateAttributes=''  IntegratorStateMustResolveToSignalObject=off  IntegratorRTWStateStorageClass=Auto  FilterContinuousStateAttributes=''  FilterStateMustResolveToSignalObject=off  FilterRTWStateStorageClass=Auto  ParallelPVariant=InternalParameters  IdealPVariant=Disabled  IVariant=InternalParameters  DVariant=InternalParameters  IntegratorVariant=Discrete  SatVariant=Enabled  AWVariant=BackCalculation  PCopyVariant=Disabled  TRVariant=Enabled  FdbkBlocksVariant=Forward  IdealPFdbkVariant=Disabled  SatFdbkVariant=Disabled  DerivativeFilterVariant=ForwardEulerFilter  NVariant=InternalParameters  NCopyVariant=Disabled  FilterICVariant=ExternalICs  IntegratorICVariant=ExternalICs  ExternalResetVariant=ExternalReset  TRSumVariant=TrackingMode  SumFdbkVariant=Disabled  SumVariant=Sum_PID  TsampFilterVariant=InternalTs  TsampNgainVariant=Passthrough  TsampIntegralVariant=Disabled_SignalSpec  ExternalSaturationOutDataTypeStr=Inherit: Same as second input  DerivativeSourceVariant=ErrorSignal  PreIntVariant=InternalPreInt
  Product : Product
  Sum3 : Sum  Inputs=|+-
  TorqueAllocator : MATLAB Function  TreatAsAtomicUnit=on  SystemSampleTime=0.05
  e_yaw * TVC_weight : Product  Inputs=**
  T_TVC_RL : Outport
  T_TVC_RR : Outport  Port=2
  wires:
  Throttle_%/1 -> Gain/1
  PID Controller/1 -> MATLAB Function/1(dMz)  "dMz"
  Product/1 -> TorqueAllocator/1(T_req)  "T_req"
  Sum3/1 -> MATLAB Function1/1(dT_act)  "dT_act"
  MATLAB Function1/1(dMz_act) -> PID Controller/5, Memory/1  "dMz_act"
  T_RL_act/1 -> Sum3/1
  T_RR_act/1 -> Sum3/2
  MATLAB Function/1(dT) -> TorqueAllocator/2(dT)  "dT"
  TorqueAllocator/1(T_RL_cmd) -> T_TVC_RL/1
  TorqueAllocator/2(T_RR_cmd) -> T_TVC_RR/1
  Der_RL/1 -> TorqueAllocator/3(derating_L)
  Der_RR/1 -> TorqueAllocator/4(derating_R)
  Constant/1 -> PID Controller/4
  Memory/1 -> PID Controller/3
  e_yaw/1 -> e_yaw * TVC_weight/1
  W/1 -> e_yaw * TVC_weight/2, Compare To Constant/1
  Compare To Constant/1 -> PID Controller/2
  e_yaw * TVC_weight/1 -> PID Controller/1
  D/1 -> TorqueAllocator/5(D)
  Max_Torque/1 -> Product/1
  Gain/1 -> Product/2  "T_req"

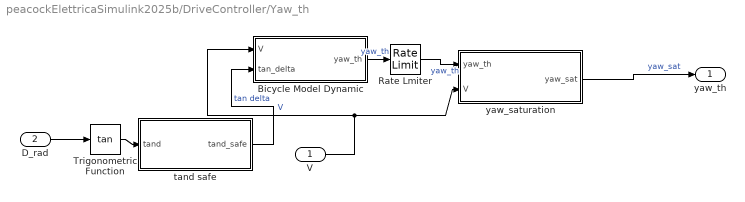
== system peacockElettricaSimulink2025b/DriveController/Yaw_th ==
  V : Inport
  D_rad : Inport  Port=2
  Bicycle Model Dynamic : MATLAB Function  TreatAsAtomicUnit=on
  Rate Lmiter : RateLimiter  SampleTimeMode=inherited
  Trigonometric Function : Trigonometry  Operator=tan
  tand safe : MATLAB Function  TreatAsAtomicUnit=on
  yaw_saturation : MATLAB Function  TreatAsAtomicUnit=on
  yaw_th : Outport
  wires:
  tand safe/1(tand_safe) -> Bicycle Model Dynamic/2(tan_delta)  "tan delta"
  Trigonometric Function/1 -> tand safe/1(tand)
  Bicycle Model Dynamic/1(yaw_th) -> Rate Lmiter/1  "yaw_th"
  V/1 -> yaw_saturation/2(V), Bicycle Model Dynamic/1(V)  "V"
  D_rad/1 -> Trigonometric Function/1
  Rate Lmiter/1 -> yaw_saturation/1(yaw_th)  "yaw_th"
  yaw_saturation/1(yaw_sat) -> yaw_th/1  "yaw_sat"

== matlab function peacockElettricaSimulink2025b/G_motor_RR/MATLAB Function ==
  data: T_thermal input; T_req input; derating_out output; derating_prev input; derating_on_thresh parameter
% function derating_out = fcn(T_thermal, derating_prev,T_peak, derating_on_thresh, derating_off_thresh)
%     if derating_prev == 0
%         % Se il limite termico cala troppo, attivo il flag
%         derating_out = double(T_thermal < derating_on_thresh);
%     else
%         % Resto in derating finché il limite non ha recuperato abbastanza
%         derating_out = double(T_thermal < derating_off_thresh);
%     end
% end

function derating_out = fcn(T_thermal, T_req, derating_prev,derating_on_thresh)

if derating_prev == 0
    % Se NON sono in derating, controllo se devo entrarci
    if T_thermal < derating_on_thresh
        derating_out = 1;
    else
        derating_out = 0;
    end
else
    if T_req <= 1 % Uso un piccolo margine invece di 0 spaccato per robustezza numerica
        derating_out = 0; % Esco dal derating
    else
        derating_out = 1; % Mantengo il derating
    end
end
end

== matlab function peacockElettricaSimulink2025b/DriveController/Yaw_th/tand safe ==
  data: tand input; tand_safe output; angle_limit parameter
% function tand_safe = fcn(tand)
%     tand_safe = sign(tand) * max(abs(tand), tan(2*pi/180));
% end
function tand_safe = fcn(tand,angle_limit)
    soglia = tan(angle_limit*pi/180);  % 2° 
    
    if abs(tand) < soglia
        tand_safe = 0;  % TV disattivato sotto soglia
    else
        tand_safe = tand;  % passa il valore reale senza clamp
    end
end

== matlab function peacockElettricaSimulink2025b/DriveController/Yaw_th/yaw_saturation ==
  data: yaw_th input; yaw_sat output; V input; mu parameter; g parameter
function yaw_sat = fcn(yaw_th, V,mu, g)
    V_calc = max(V, 0.5);
    
    yaw_max_abs = (mu * g) / V_calc;
    yaw_sat = sign(yaw_th) * min(abs(yaw_th), yaw_max_abs);
end

== matlab function peacockElettricaSimulink2025b/DriveController/SRC/MATLAB Function ==
  data: enable input; T_cut_RL output; Delta_T_raw input
function T_cut_RL = fcn(enable, Delta_T_raw)
    T_cut_RL = enable * Delta_T_raw;
end

== matlab function peacockElettricaSimulink2025b/DriveController/SRC/MATLAB Function1 ==
  data: enable input; T_cut_RR output; Delta_T_raw input
function T_cut_RR = fcn(enable, Delta_T_raw)
    T_cut_RR = enable * Delta_T_raw;
end

== matlab function peacockElettricaSimulink2025b/MATLAB Function1 ==
  data: Vx input; Vx_hub output; Vy input; yaw input; delta_L input; delta_R input; Vy_hub output; track_width_f parameter; track_width_r parameter; l_f parameter; l_r parameter
function [Vx_hub, Vy_hub] = wheel_kinematics(Vx, Vy, yaw, delta_L, delta_R, track_width_f, track_width_r, l_f, l_r)
% Trasforma le velocità del baricentro (CG) nelle velocità locali dei mozzi ruota.
%
% INPUTS:
% Vx, Vy  : Velocità longitudinali e laterali del veicolo (CG) [m/s]
% yaw       : Velocità di imbardata (Yaw rate) [rad/s]
% delta_L : Angolo di sterzo ruota anteriore sinistra [rad]
% delta_R : Angolo di sterzo ruota anteriore destra [rad]
% l_f, l_r: Distanza baricentro - asse anteriore/posteriore [m]
% track_width_f, track_width_r: Carreggiata (Track width) anteriore/posteriore [m]
%
% OUTPUTS:
% Vx_hub  : Vettore [FL, FR, RL, RR] delle velocità longitudinali dei mozzi [m/s]
% Vy_hub  : Vettore [FL, FR, RL, RR] delle velocità laterali dei mozzi [m/s]

    %% 1. Velocità nel sistema di riferimento del telaio (non ruotate)
    % Anteriore Sinistra (Front Left)
    V_xf_FL = Vx - (yaw * track_width_f / 2);
    V_yf_FL = Vy + (yaw * l_f);
    
    % Anteriore Destra (Front Right)
    V_xf_FR = Vx + (yaw * track_width_f / 2);
    V_yf_FR = Vy + (yaw * l_f);
    
    % Posteriore Sinistra (Rear Left)
    V_xr_RL = Vx - (yaw * track_width_r / 2);
    V_yr_RL = Vy - (yaw * l_r);
    
    % Posteriore Destra (Rear Right)
    V_xr_RR = Vx + (yaw * track_width_r / 2);
    V_yr_RR = Vy - (yaw * l_r);

    %% 2. Rotazione nel sistema di riferimento della gomma (tramite angolo di sterzo)
    % Le ruote anteriori sono sterzanti
    Vx_FL =  V_xf_FL * cos(delta_L) + V_yf_FL * sin(delta_L);
    Vy_FL = -V_xf_FL * sin(delta_L) + V_yf_FL * cos(delta_L);
    
    Vx_FR =  V_xf_FR * cos(delta_R) + V_yf_FR * sin(delta_R);
    Vy_FR = -V_xf_FR * sin(delta_R) + V_yf_FR * cos(delta_R);
    
    % Le ruote posteriori solitamente non sterzano (delta = 0, quindi cos(0)=1, sin(0)=0)
    Vx_RL = V_xr_RL;
    Vy_RL = V_yr_RL;
    
    Vx_RR = V_xr_RR;
    Vy_RR = V_yr_RR;

    Vx_hub = [Vx_FL; Vx_FR; Vx_RL; Vx_RR];
    Vy_hub = [Vy_FL; Vy_FR; Vy_RL; Vy_RR];
end

== matlab function peacockElettricaSimulink2025b/DriveController/MATLAB Function ==
  settings: updateMethod=DISCRETE
  data: throttle_pct input; T_regen_RL output; n_motorRL input; n_motorRR input; V input; T_regen_RR output; regen_active output; Ts parameter; regen_T_max parameter; regen_pedal_thr parameter; regen_speed_min_rpm parameter; regen_speed_crit_rpm parameter; regen_I_peak_A parameter; regen_I_cont_A parameter; regen_I_peak_dur_s parameter; regen_P_batt_max_W parameter; V_dc parameter
function [T_regen_RL, T_regen_RR, regen_active] = regen_fcn( ...
        throttle_pct, n_motorRL, n_motorRR, V, Ts, ...
regen_T_max, regen_pedal_thr, regen_speed_min_rpm, regen_speed_crit_rpm, ...
regen_I_peak_A, regen_I_cont_A, regen_I_peak_dur_s, ...
regen_P_batt_max_W, V_dc)
%REGEN_FCN  Logica di frenata rigenerativa per MATLAB Function block.
%
%  Specchio del codice STM32 (Regen.c) adattato a Simulink discreto.
%  Usare come MATLAB Function block nel DriveController.
%
%  Vincolo BMS (TOTALE su 2 motori):
%    Peak:  regen_I_peak_A [A] per i primi regen_I_peak_dur_s [s]
%    Cont:  regen_I_cont_A [A] dopo la finestra peak
%  Il timer si azzera quando il pilota NON sta richiedendo regen.
%
%  Stage 1 – Coppia pedal-dipendente (lineare)
%  Stage 2 – Fade-out a bassa velocità
%  Stage 3 – Limite di potenza batteria
%  Stage 5 – Limite corrente BMS (peak/cont con timer discreto)
%
%  Stage 4 (derating tensione DC) omesso: modello non ha V_dc dinamico.
%
%  OUTPUT:
%    T_regen_RL/RR : coppia regen per motore [Nm], negativa o zero
%    regen_active  : flag 0/1

    persistent t_elapsed_s;
    if isempty(t_elapsed_s)
        t_elapsed_s = 0.0;
    end

    speed_avg_rpm = (abs(n_motorRL) + abs(n_motorRR)) * 0.5;

    % ---- condizione di abilitazione regen (con isteresi velocità) -------
    % Entra se:  pedal < soglia  E  speed > crit  E  veicolo in moto
    % Reset se:  pedal >= soglia  O  speed < crit  O  veicolo fermo
    should_regen = (throttle_pct <= regen_pedal_thr) && ...
                   (speed_avg_rpm > regen_speed_crit_rpm) && ...
                   (V > 0.5);

    if ~should_regen
        % Azzeramento timer (prossima attivazione riparte da zero)
        t_elapsed_s = 0.0;
        T_regen_RL  = 0.0;
        T_regen_RR  = 0.0;
        regen_active = 0.0;
        return;
    end

    % ---- timer discreto (equivalente a HAL_GetTick diff) ----------------
    t_elapsed_s = t_elapsed_s + Ts;

    % ---- Stage 1: coppia pedal-dipendente [Nm, negativa] ----------------
    % T = -T_max * (1 - pedal / soglia)
    % pedal = 0  → T = -T_max   (regen massima)
    % pedal = soglia → T = 0    (nessuna regen)
    pedal_norm = throttle_pct / regen_pedal_thr;
    T_s1 = -regen_T_max * (1.0 - pedal_norm);

    % ---- Stage 2: fade-out velocità [fattore k_vel ∈ [0,1]] ------------
    % k_vel = 1           se speed >= speed_min
    % k_vel = speed/min   se speed <  speed_min  (crit < speed < min)
    if speed_avg_rpm >= regen_speed_min_rpm
        k_vel = 1.0;
    else
        k_vel = speed_avg_rpm / regen_speed_min_rpm;
    end
    T_s2 = T_s1 * k_vel;

    % ---- Stage 3: limite potenza batteria (per motore = totale/2) -------
    % |T| <= P_max_per_mot / omega
    omega_rad_s = (2.0 * pi * speed_avg_rpm) / 60.0;
    omega_safe  = max(omega_rad_s, 1.0);          % evita div/0 a bassa velocità
    T_P_lim     = (regen_P_batt_max_W * 0.5) / omega_safe;
    T_s3        = max(T_s2, -T_P_lim);            % T_s2 è negativo → clamp inferiore

    % ---- Stage 5: limite corrente BMS con finestra peak/cont ------------
    % Corrente TOTALE / 2 motori = corrente per motore
    % T_lim = (I_lim_per_mot * V_dc) / omega
    if t_elapsed_s < regen_I_peak_dur_s
        I_lim_per_mot = regen_I_peak_A * 0.5;    % 21/2 = 10.5 A
    else
        I_lim_per_mot = regen_I_cont_A  * 0.5;   % 14/2 = 7.0 A
    end
    T_I_lim = (I_lim_per_mot * V_dc) / omega_safe;
    T_final = max(T_s3, -T_I_lim);               % clamp (T_s3 negativo)

    % ---- output simmetrico sui due motori --------------------------------
    T_regen_RL  = T_final;
    T_regen_RR  = T_final;
    regen_active = 1.0;
end

== matlab function peacockElettricaSimulink2025b/DriveController/TVC/MATLAB Function ==
  data: dMz input; dT output; R_wheel parameter; track_width parameter
function dT = fcn(dMz,R_wheel, track_width)
    dT = dMz * R_wheel / track_width;
end

== matlab function peacockElettricaSimulink2025b/DriveController/Yaw_th/Bicycle Model Dynamic ==
  data: V input; yaw_th output; tan_delta input; wheelbase parameter; Kus parameter
function yaw_th = fcn(V,tan_delta,wheelbase,Kus)
% L = 1.55; %passo veicolo [m]
% yaw_th = (V / L) * tand;
%
  
yaw_th = (V / wheelbase) * tan_delta / (1 + Kus * V^2);



end

== matlab function peacockElettricaSimulink2025b/DriveController/TVC/MATLAB Function1 ==
  data: dT_act input; dMz_act output; track_width parameter; R_wheel parameter
function dMz_act = fcn(dT_act,track_width, R_wheel)


dMz_act = dT_act * track_width / (2*R_wheel);
%dMz_act = -(dT_act * w / (2*Rw)); 

end

== matlab function peacockElettricaSimulink2025b/MATLAB Function ==
  data: Vx input; V output; Vy input
function V = fcn(Vx,Vy)

V = (Vx^2 + Vy^2)^0.5;

== stateflow chart peacockElettricaSimulink2025b/DriveController/Mode Manager ==
  state IDLE_
    entry:
    TVC_Target_Weight = 0;
  state SLC_
    entry: TVC_Target_Weight = 0;
  state TVC_
    entry: TVC_Target_Weight = 1;
  (default) -> IDLE_
  SLC_ -> IDLE_ [order 2] : [Throttle < 2 && V <= 0.5]
  TVC_ -> IDLE_ [order 2] : [brake > 0 || V <= 0.5]
  IDLE_ -> SLC_ : [Throttle > tvc_throttle_on && brake == 0]
  TVC_ -> SLC_ [order 1] : [abs(D) < tvc_D_thresh_off && abs(YawError) < tvc_yaw_thresh_off || V < tvc_V_off ]
  SLC_ -> TVC_ [order 1] : [(abs(D) > tvc_D_thresh || abs(YawError) > tvc_yaw_thresh) && V > tvc_V_on && brake == 0]
  data: TVC_Target_Weight output; V input; D input; Throttle input; YawError input; brake input; tvc_D_thresh parameter; tvc_yaw_thresh parameter; tvc_yaw_thresh_off parameter; tvc_throttle_on parameter; tvc_V_on parameter; tvc_V_off parameter; tvc_D_thresh_off parameter

== matlab function peacockElettricaSimulink2025b/G_motor_RL/MATLAB Function ==
  data: T_thermal input; T_req input; derating_out output; derating_prev input; derating_on_thresh parameter
% function derating_out = fcn(T_thermal, derating_prev,T_peak, derating_on_thresh, derating_off_thresh)
%     if derating_prev == 0
%         % Se il limite termico cala troppo, attivo il flag
%         derating_out = double(T_thermal < derating_on_thresh);
%     else
%         % Resto in derating finché il limite non ha recuperato abbastanza
%         derating_out = double(T_thermal < derating_off_thresh);
%     end
% end

function derating_out = fcn(T_thermal, T_req, derating_prev,derating_on_thresh)

if derating_prev == 0
    % Se NON sono in derating, controllo se devo entrarci
    if T_thermal < derating_on_thresh
        derating_out = 1;
    else
        derating_out = 0;
    end
else
    if T_req <= 1 % Uso un piccolo margine invece di 0 spaccato per robustezza numerica
        derating_out = 0; % Esco dal derating
    else
        derating_out = 1; % Mantengo il derating
    end
end
end
